simulink model "HW7_SIP_tmrpns_2"  (Simulink 8.6)
settings: Solver=ode3  StartTime=0.0  StopTime=40  FixedStep=0.001  RelTol=1e-3
values from neighbouring files (symbols this model uses):
  F = [-9-wn^2  0.6-2*ze*wn]    [HW7_SIP_1.m]
  x10 = x10_deg*3.1416/180    (= 0.2618)    [HW7_SIP_1.m]
settings Model: Creator=BC  LastModifiedBy=bcc88  ExtModeTrigMode=oneshot  ExtModeArmWhenConnect=off
settings DataIOCC: LimitDataPoints=off
settings OptimizationCC: BlockReduction=off  BooleanDataType=off  InitFltsAndDblsToZero=on
settings DebuggingCC: SaveWithParameterizedLinksMsg=none  SignalResolutionControl=TryResolveAllWithWarning  SolverPrmCheckMsg=none  MultiTaskDSMMsg=warning  MultiTaskCondExecSysMsg=none  FcnCallInpInsideContextMsg=UseLocalSettings
settings HardwareCC: TargetUnknown=on
settings GRTTargetCC: TargetFcnLib=ansi_tfl_tmw.mat  GeneratePreprocessorConditionals=Use local settings

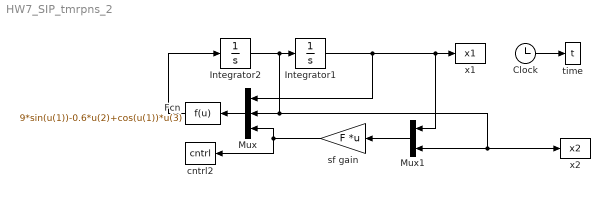
== system HW7_SIP_tmrpns_2 ==
  Clock : Clock
  Fcn : Fcn  Expr=9*sin(u(1))-0.6*u(2)+cos(u(1))*u(3)
  Integrator1 : Integrator  InitialCondition=x10
  Integrator2 : Integrator
  Mux : Mux  Inputs=3
  Mux1 : Mux  Inputs=2
  cntrl2 : ToWorkspace  VariableName=cntrl  SampleTime=-1
  sf gain : Gain  Gain=F  Multiplication=Matrix(K*u)
  time : ToWorkspace  VariableName=t  SampleTime=-1
  x1 : ToWorkspace  VariableName=x1  SampleTime=-1
  x2 : ToWorkspace  VariableName=x2  SampleTime=-1
  wires:
  Fcn/1 -> Integrator2/1
  Integrator2/1 -> Integrator1/1, Mux1/2, x2/1, Mux/2
  Clock/1 -> time/1
  Mux/1 -> Fcn/1
  Mux1/1 -> sf gain/1
  sf gain/1 -> cntrl2/1, Mux/3
  Integrator1/1 -> Mux/1, x1/1, Mux1/1
